simulink model "partage_reglesIHM"  (Simulink 7.5)
settings: Solver=ode45  StartTime=0.0  StopTime=10.0  RelTol=1e-3
settings Model: Creator=paris  LastModifiedBy=paris

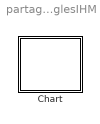
== system partage_reglesIHM ==
  Chart : Stateflow chart  TreatAsAtomicUnit=on

== stateflow chart Chart ==
  state Regles_Decisinnelles_Interaction_Homme_Machine
    state Conduite_Dans_Voie
    state Aide_Requise
      state Aide_Maintien_Voie
      state Correction_Habitudes
    state Ne_Pas_Entraver_Activite
      state Legitime_Critique
      state Legitime_NonCritique
      (junction 11) -> Legitime_Critique [order 4]
      (default) -> (junction 11)
      (junction 11) -> Legitime_NonCritique [order 3] : [ml.lateralisation_SV==-1 && ml.trafic_oppose==0]
      (junction 11) -> Legitime_NonCritique [order 2] : [ml.lateralisation_SV==1 && ml.type_accotement==68]
      (junction 11) -> Legitime_NonCritique [order 1] : [ml.lateralisation_SV==1 && ml.type_accotement==69]
    Regles_Decisinnelles_Interaction_Homme_Machine -> Ne_Pas_Entraver_Activite [order 4] : [in(Jugement_Adequation_Comportement.Sortie_Voie_Legitime)]
    Regles_Decisinnelles_Interaction_Homme_Machine -> Conduite_Dans_Voie [order 2] : [in(Jugement_Adequation_Comportement.Conduite_Dans_Voie)]
    Regles_Decisinnelles_Interaction_Homme_Machine -> Aide_Maintien_Voie [order 1] : [in(Jugement_Adequation_Comportement.Defaut_Maitrise)]
    Regles_Decisinnelles_Interaction_Homme_Machine -> Correction_Habitudes [order 3] : [in(Jugement_Adequation_Comportement.Defaut_Maitrise)]
    (default) -> Conduite_Dans_Voie
